simulink model "distributed_UIO_4nodes_switching"  (R2021a)
settings: Solver=VariableStepAuto  StartTime=0.0  StopTime=50  FixedStep=1e-6  RelTol=1e-6
values from neighbouring files (symbols this model uses):
  A = [0,1,0,0,0,0,0,0 ... (first row only)    [UIO_parameters_4nodes_invertedpendulum.m]    (also in UIO_parameters_4nodes_perturbation.m = Xi - diag(sum(Xi,2)); UIO_parameters_4nodes_room_T.m = Xi - diag(sum(Xi,2)); UIO_parameters_4nodes_unknowninputs_directed.m = Xi - diag(sum(Xi,2)); UIO_parameters_4nodes_unknowninputs_switching.m = Xi - diag(sum(Xi,2)))
  B1 = B(:,1)    [UIO_parameters_4nodes_invertedpendulum.m]    (also in UIO_parameters_4nodes_perturbation.m; UIO_parameters_4nodes_room_T.m; UIO_parameters_4nodes_unknowninputs_directed.m; UIO_parameters_4nodes_unknowninputs_switching.m)
  B2 = B(:,2)    [UIO_parameters_4nodes_invertedpendulum.m]    (also in UIO_parameters_4nodes_perturbation.m; UIO_parameters_4nodes_room_T.m; UIO_parameters_4nodes_unknowninputs_directed.m; UIO_parameters_4nodes_unknowninputs_switching.m)
  B3 = B(:,3)    [UIO_parameters_4nodes_invertedpendulum.m]    (also in UIO_parameters_4nodes_perturbation.m; UIO_parameters_4nodes_room_T.m; UIO_parameters_4nodes_unknowninputs_directed.m; UIO_parameters_4nodes_unknowninputs_switching.m)
  C1 = [0,0,0,1,0,0,0,0 ... (first row only)    [UIO_parameters_4nodes_invertedpendulum.m]    (also in UIO_parameters_4nodes_perturbation.m = [0,0,0,0,1,0,0,0,0; UIO_parameters_4nodes_room_T.m = [0,0,0,0,1,0,0,0,0; UIO_parameters_4nodes_unknowninputs_directed.m = [0,0,0,0,1,0,0,0,0; UIO_parameters_4nodes_unknowninputs_switching.m = [0,0,0,0,1,0,0,0,0)
  C2 = [0,1,0,0,0,0,0,0 ... (first row only)    [UIO_parameters_4nodes_invertedpendulum.m]    (also in UIO_parameters_4nodes_perturbation.m = [0,1,0,0,0,0,0,0,0; UIO_parameters_4nodes_room_T.m = [0,1,0,0,0,0,0,0,0; UIO_parameters_4nodes_unknowninputs_directed.m = [0,1,0,0,0,0,0,0,0; UIO_parameters_4nodes_unknowninputs_switching.m = [0,1,0,0,0,0,0,0,0)
  C3 = [0,0,0,1,0,0,0,0 ... (first row only)    [UIO_parameters_4nodes_invertedpendulum.m]    (also in UIO_parameters_4nodes_perturbation.m = [0,1,0,0,0,0,0,0,0; UIO_parameters_4nodes_room_T.m = [0,1,0,0,0,0,0,0,0; UIO_parameters_4nodes_unknowninputs_directed.m = [0,1,0,0,0,0,0,0,0; UIO_parameters_4nodes_unknowninputs_switching.m = [0,1,0,0,0,0,0,0,0)
  C4 = [0,1,0,0,0,0,0,0 ... (first row only)    [UIO_parameters_4nodes_invertedpendulum.m]    (also in UIO_parameters_4nodes_perturbation.m = [0,1,0,0,0,0,0,0,0; UIO_parameters_4nodes_room_T.m = [0,1,0,0,0,0,0,0,0; UIO_parameters_4nodes_unknowninputs_directed.m = [0,1,0,0,0,0,0,0,0; UIO_parameters_4nodes_unknowninputs_switching.m = [0,1,0,0,0,0,0,0,0)
  chi = norm(Lambda + Lambda_P'*(-sum_Lambda)^(-1)*Lambda_P)/(2*lambda_2)+1    [UIO_parameters_4nodes_invertedpendulum.m]    (also in UIO_parameters_4nodes_perturbation.m = norm(Lambda + Lambda_P'*(-sum_Lambda)^(-1)*Lambda_P)/(2*lamb; UIO_parameters_4nodes_room_T.m = norm(Lambda + Lambda_P'*(-sum_Lambda)^(-1)*Lambda_P)/(2*lamb; UIO_parameters_4nodes_unknowninputs_directed.m = norm(Lambda + Lambda_P'*(-sum_Lambda)^(-1)*Lambda_P)/hatLap2; UIO_parameters_4nodes_unknowninputs_switching.m = norm(Lambda + Lambda_P'*(-sum_Lambda)^(-1)*Lambda_P)/(2*CN)+)
  D = B(:,4)    [UIO_parameters_4nodes_invertedpendulum.m]    (also in UIO_parameters_4nodes_perturbation.m; UIO_parameters_4nodes_room_T.m; UIO_parameters_4nodes_unknowninputs_directed.m; UIO_parameters_4nodes_unknowninputs_switching.m)
  F = place(A,[B1,B2,B3],-1*[0.1 0.2 0.3 0.4 0.5 0.6 0.7 0.8])    [UIO_parameters_4nodes_invertedpendulum.m]    (also in UIO_parameters_4nodes_perturbation.m = place(A,[B1,B2,B3],-1*[0.1 0.2 0.3 0.4 0.5 0.6 0.7 0.8 0.9]); UIO_parameters_4nodes_room_T.m = place(A,[B1,B2,B3],-1*[0.1 0.2 0.3 0.4 0.5 0.6 0.7 0.8 0.9]); UIO_parameters_4nodes_unknowninputs_directed.m = place(A,[B1,B2,B3],-1*[0.1 0.2 0.3 0.4 0.5 0.6 0.7 0.8 0.9]); UIO_parameters_4nodes_unknowninputs_switching.m = place(A,[B1,B2,B3],-1*[0.1 0.2 0.3 0.4 0.5 0.6 0.7 0.8 0.9]))
  H1 = U1 + Y1*V1    [UIO_parameters_4nodes_invertedpendulum.m]    (also in UIO_parameters_4nodes_perturbation.m; UIO_parameters_4nodes_room_T.m; UIO_parameters_4nodes_unknowninputs_directed.m; UIO_parameters_4nodes_unknowninputs_switching.m)
  H2 = U2 + Y2*V2    [UIO_parameters_4nodes_invertedpendulum.m]    (also in UIO_parameters_4nodes_perturbation.m; UIO_parameters_4nodes_room_T.m; UIO_parameters_4nodes_unknowninputs_directed.m; UIO_parameters_4nodes_unknowninputs_switching.m)
  H3 = U3 + Y3*V3    [UIO_parameters_4nodes_invertedpendulum.m]    (also in UIO_parameters_4nodes_perturbation.m; UIO_parameters_4nodes_room_T.m; UIO_parameters_4nodes_unknowninputs_directed.m; UIO_parameters_4nodes_unknowninputs_switching.m)
  H4 = U4 + Y4*V4    [UIO_parameters_4nodes_invertedpendulum.m]    (also in UIO_parameters_4nodes_perturbation.m; UIO_parameters_4nodes_room_T.m; UIO_parameters_4nodes_unknowninputs_directed.m; UIO_parameters_4nodes_unknowninputs_switching.m)
  L1 = K1 + N1*H1    [UIO_parameters_4nodes_invertedpendulum.m]    (also in UIO_parameters_4nodes_perturbation.m; UIO_parameters_4nodes_room_T.m; UIO_parameters_4nodes_unknowninputs_directed.m; UIO_parameters_4nodes_unknowninputs_switching.m)
  L2 = K2 + N2*H2    [UIO_parameters_4nodes_invertedpendulum.m]    (also in UIO_parameters_4nodes_perturbation.m; UIO_parameters_4nodes_room_T.m; UIO_parameters_4nodes_unknowninputs_directed.m; UIO_parameters_4nodes_unknowninputs_switching.m)
  L3 = K3 + N3*H3    [UIO_parameters_4nodes_invertedpendulum.m]    (also in UIO_parameters_4nodes_perturbation.m; UIO_parameters_4nodes_room_T.m; UIO_parameters_4nodes_unknowninputs_directed.m; UIO_parameters_4nodes_unknowninputs_switching.m)
  L4 = K4 + N4*H4    [UIO_parameters_4nodes_invertedpendulum.m]    (also in UIO_parameters_4nodes_perturbation.m; UIO_parameters_4nodes_room_T.m; UIO_parameters_4nodes_unknowninputs_directed.m; UIO_parameters_4nodes_unknowninputs_switching.m)
  M1 = eye(n) - H1*C1    [UIO_parameters_4nodes_invertedpendulum.m]    (also in UIO_parameters_4nodes_perturbation.m; UIO_parameters_4nodes_room_T.m; UIO_parameters_4nodes_unknowninputs_directed.m; UIO_parameters_4nodes_unknowninputs_switching.m)
  M2 = eye(n) - H2*C2    [UIO_parameters_4nodes_invertedpendulum.m]    (also in UIO_parameters_4nodes_perturbation.m; UIO_parameters_4nodes_room_T.m; UIO_parameters_4nodes_unknowninputs_directed.m; UIO_parameters_4nodes_unknowninputs_switching.m)
  M3 = eye(n) - H3*C3    [UIO_parameters_4nodes_invertedpendulum.m]    (also in UIO_parameters_4nodes_perturbation.m; UIO_parameters_4nodes_room_T.m; UIO_parameters_4nodes_unknowninputs_directed.m; UIO_parameters_4nodes_unknowninputs_switching.m)
  N1 = M1*A - K1*C1    [UIO_parameters_4nodes_invertedpendulum.m]    (also in UIO_parameters_4nodes_perturbation.m; UIO_parameters_4nodes_room_T.m; UIO_parameters_4nodes_unknowninputs_directed.m; UIO_parameters_4nodes_unknowninputs_switching.m)
  N2 = M2*A - K2*C2    [UIO_parameters_4nodes_invertedpendulum.m]    (also in UIO_parameters_4nodes_perturbation.m; UIO_parameters_4nodes_room_T.m; UIO_parameters_4nodes_unknowninputs_directed.m; UIO_parameters_4nodes_unknowninputs_switching.m)
  N3 = M3*A - K3*C3    [UIO_parameters_4nodes_invertedpendulum.m]    (also in UIO_parameters_4nodes_perturbation.m; UIO_parameters_4nodes_room_T.m; UIO_parameters_4nodes_unknowninputs_directed.m; UIO_parameters_4nodes_unknowninputs_switching.m)
  N4 = M4*A - K4*C4    [UIO_parameters_4nodes_invertedpendulum.m]    (also in UIO_parameters_4nodes_perturbation.m; UIO_parameters_4nodes_room_T.m; UIO_parameters_4nodes_unknowninputs_directed.m; UIO_parameters_4nodes_unknowninputs_switching.m)
  P1 = [0.1 -2.74787163193e-21 -6.58900207734e-22 1.45624208773e-22 2.15066555276e-36 2.0153156439e-36 -1.50571830434e-21 -1.03899300906e-23 2.18840927595e-36 -2.74787163193e-21 0.1 -2.05830389854e-21 ... (81 elements, 9x9)]    [paras_T.mat]
  P2 = [0.1 7.3646299452e-36 -1.12803244841e-21 -8.66266671459e-22 7.23314160582e-22 7.39056861945e-36 -8.2159683555e-21 6.09745804933e-22 7.34683360427e-36 7.3646299452e-36 0.1 1.40040566631e-35 ... (81 elements, 9x9)]    [paras_T.mat]
  P3 = [0.1 -2.18794371664e-37 3.91368207909e-22 3.65670921511e-22 -2.55025634775e-37 -1.42860183838e-23 2.63558676e-21 -2.22685468476e-22 -3.11406679403e-37 -2.18794371664e-37 0.1 -8.43108395867e-38 ... (81 elements, 9x9)]    [paras_T.mat]
  P4 = [0.1 2.36535861574e-35 -1.59743131024e-21 -1.41330471892e-21 2.3619901104e-35 2.36062716781e-35 -1.18359612306e-20 7.3423642543e-22 2.36207112865e-35 2.36535861574e-35 0.1 3.81668075057e-35 ... (81 elements, 9x9)]    [paras_T.mat]
  x0 = -30/180*pi+2*30/180*pi*rand(n,1)    [UIO_parameters_4nodes_invertedpendulum.m]    (also in UIO_parameters_4nodes_perturbation.m = [15.8;27.5;7.4;8.1;11.2;23.2;25.3;23.2;18.3]; UIO_parameters_4nodes_room_T.m = [15.8;27.5;7.4;8.1;11.2;23.2;25.3;23.2;18.3]; UIO_parameters_4nodes_unknowninputs_directed.m = [15.8;27.5;7.4;8.1;11.2;23.2;25.3;23.2;18.3]; UIO_parameters_4nodes_unknowninputs_switching.m = [15.8;27.5;7.4;8.1;11.2;23.2;25.3;23.2;18.3])
  xset = 18*ones(n,1)    [UIO_parameters_4nodes_perturbation.m]    (also in UIO_parameters_4nodes_room_T.m; UIO_parameters_4nodes_unknowninputs_directed.m; UIO_parameters_4nodes_unknowninputs_switching.m; paras_T.mat = [18 18 18 18 18 18 18 18 18])
libraries: simulink x1
settings Model: Creator=gy116  LastModifiedBy=gy116
settings SolverCC: AlgebraicLoopSolver=LineSearch
settings DataIOCC: ReturnWorkspaceOutputs=off
settings DebuggingCC: SFMachineParentedDataDiag=warning  ArithmeticOperatorsInVariantConditions=warning
settings SFSimCC: SimUseLocalCustomCode=off  CustomCodeUndefinedFunction=UseInterfaceOnly
settings RTWCC: RTWUseLocalCustomCode=off
settings CodeAppCC: StateflowObjectComments=on

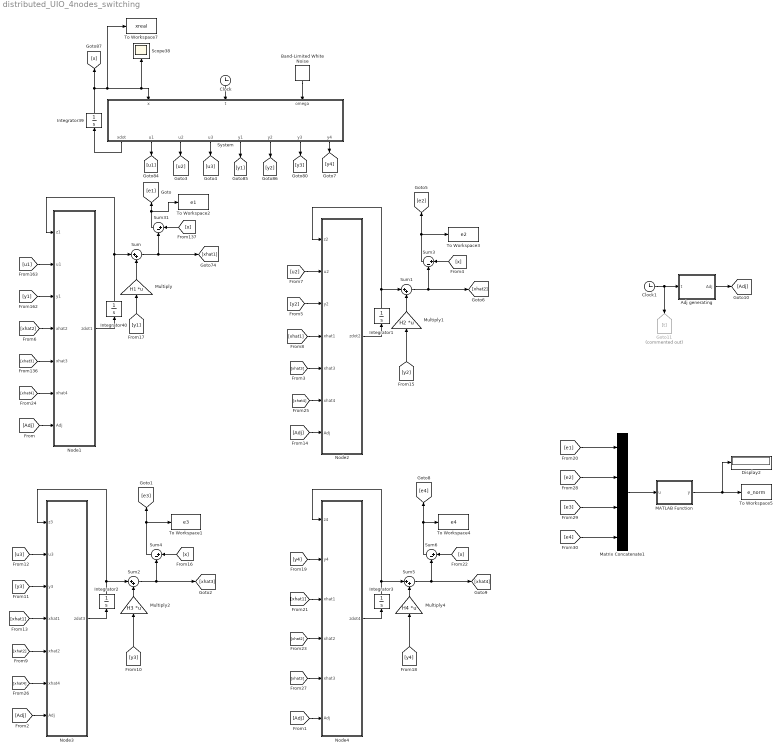
== system distributed_UIO_4nodes_switching ==
  Adj generating : MATLAB Function  TreatAsAtomicUnit=on
  Band-Limited White Noise : simulink/Sources/Band-Limited White Noise  Cov=[1]  Ts=0.1  seed=[23341]
  Clock : Clock
  Clock1 : Clock
  Display2 : Display
  Goto11 : Goto  Commented=on  GotoTag=t
  Integrator{1..3,40} (4 alike) : Integrator  InitialCondition=0*x0
  Integrator39 : Integrator  InitialCondition=x0
  MATLAB Function : MATLAB Function  TreatAsAtomicUnit=on
  Matrix Concatenate1 : Concatenate  NumInputs=4  ConcatenateDimension=2
  Multiply : Gain  Gain=H1  Multiplication=Matrix(K*u) (u vector)
  Multiply1 : Gain  Gain=H2  Multiplication=Matrix(K*u) (u vector)
  Multiply2 : Gain  Gain=H3  Multiplication=Matrix(K*u) (u vector)
  Multiply4 : Gain  Gain=H4  Multiplication=Matrix(K*u) (u vector)
  Node1 : MATLAB Function  TreatAsAtomicUnit=on
  Node2 : MATLAB Function  TreatAsAtomicUnit=on
  Node3 : MATLAB Function  TreatAsAtomicUnit=on
  Node4 : MATLAB Function  TreatAsAtomicUnit=on
  Scope38 : Scope
  Sum{,1..2,5} (4 alike) : Sum  Inputs=|++
  Sum{3..4,6,31} (4 alike) : Sum  Inputs=|+-
  System : MATLAB Function  TreatAsAtomicUnit=on
  To Workspace1 : ToWorkspace  VariableName=e3  SaveFormat=Structure With Time  SampleTime=-1
  To Workspace2 : ToWorkspace  VariableName=e1  SaveFormat=Structure With Time  SampleTime=-1
  To Workspace3 : ToWorkspace  VariableName=e2  SaveFormat=Structure With Time  SampleTime=-1
  To Workspace4 : ToWorkspace  VariableName=e4  SaveFormat=Structure With Time  SampleTime=-1
  To Workspace5 : ToWorkspace  VariableName=e_norm  SaveFormat=Structure With Time  SampleTime=-1
  To Workspace7 : ToWorkspace  VariableName=xreal  SaveFormat=Structure With Time  SampleTime=-1
  wires:
  Clock1/1 -> Adj generating/1(t), Goto11/1
  Adj generating/1(Adj) -> [Adj]
  [x] -> Sum6/1
  Integrator40/1 -> Sum/1, Node1/1(z1)
  [xhat1] -> Node3/4(xhat1)
  Sum6/1 -> To Workspace4/1, [e4]
  Multiply4/1 -> Sum5/2
  Integrator3/1 -> Sum5/1, Node4/1(z4)
  Node1/1(zdot1) -> Integrator40/1
  [y1] -> Node1/3(y1)
  Sum2/1 -> Sum4/2, [xhat3]
  [y1] -> Multiply/1
  [y3] -> Multiply2/1
  [y2] -> Multiply1/1
  Sum/1 -> Sum31/2, [xhat1]
  Node4/1(zdot4) -> Integrator3/1
  Integrator39/1 -> To Workspace7/1, System/1(x), Scope38/1, [x]
  Band-Limited White Noise/1 -> System/3(omega)
  [u3] -> Node3/2(u3)
  [y4] -> Multiply4/1
  Sum1/1 -> Sum3/2, [xhat2]
  [xhat4] -> Node2/6(xhat4)
  System/8(y4) -> [y4]
  System/5(y1) -> [y1]
  [y4] -> Node4/2(y4)
  [xhat2] -> Node4/4(xhat2)
  [xhat3] -> Node4/5(xhat3)
  Multiply1/1 -> Sum1/2
  Sum3/1 -> To Workspace3/1, [e2]
  System/1(xdot) -> Integrator39/1
  System/3(u2) -> [u2]
  Clock/1 -> System/2(t)
  [xhat2] -> Node1/4(xhat2)
  System/7(y3) -> [y3]
  [x] -> Sum31/1
  System/2(u1) -> [u1]
  Integrator1/1 -> Sum1/1, Node2/1(z2)
  [xhat4] -> Node3/6(xhat4)
  [y2] -> Node2/3(y2)
  [y3] -> Node3/3(y3)
  Integrator2/1 -> Sum2/1, Node3/1(z3)
  Sum31/1 -> To Workspace2/1, [e1]
  [xhat3] -> Node2/5(xhat3)
  [u2] -> Node2/2(u2)
  [xhat2] -> Node3/5(xhat2)
  Multiply/1 -> Sum/2
  System/6(y2) -> [y2]
  [xhat3] -> Node1/5(xhat3)
  [x] -> Sum3/1
  Node2/1(zdot2) -> Integrator1/1
  Node3/1(zdot3) -> Integrator2/1
  [x] -> Sum4/1
  [u1] -> Node1/2(u1)
  [xhat1] -> Node2/4(xhat1)
  Sum4/1 -> To Workspace1/1, [e3]
  System/4(u3) -> [u3]
  Sum5/1 -> Sum6/2, [xhat4]
  [xhat1] -> Node4/3(xhat1)
  Multiply2/1 -> Sum2/2
  [xhat4] -> Node1/6(xhat4)
  [Adj] -> Node1/7(Adj)
  [Adj] -> Node2/7(Adj)
  [Adj] -> Node3/7(Adj)
  [Adj] -> Node4/6(Adj)
  [e4] -> Matrix Concatenate1/4
  Matrix Concatenate1/1 -> MATLAB Function/1(u)
  [e1] -> Matrix Concatenate1/1
  [e3] -> Matrix Concatenate1/3
  MATLAB Function/1(y) -> Display2/1, To Workspace5/1
  [e2] -> Matrix Concatenate1/2

== matlab function distributed_UIO_4nodes_switching/MATLAB Function ==
  data: u input; y output
function y = fcn(u)

y = norm(u);

== matlab function distributed_UIO_4nodes_switching/Node1 ==
  data: z1 input; u1 input; y1 input; xhat2 input; xhat3 input; xhat4 input; zdot1 output; N1 parameter; M1 parameter; L1 parameter; P1 parameter; B1 parameter; H1 parameter; chi parameter; Adj input
function zdot1  = fcn(z1,u1,y1,xhat2,xhat3,xhat4,N1, M1, L1, P1,B1, H1, chi, Adj)

commu1 =  Adj(1,2)*(xhat2-z1-H1*y1) + Adj(1,3)*(xhat3-z1-H1*y1) + Adj(1,4)*(xhat4-z1-H1*y1);

zdot1 = N1*z1 + M1*B1*u1 + L1*y1 + chi*P1^(-1)*commu1;

== matlab function distributed_UIO_4nodes_switching/System ==
  data: x input; t input; A parameter; xdot output; u1 output; u2 output; u3 output; y1 output; y2 output; y3 output; B1 parameter; B2 parameter; B3 parameter; C2 parameter; C3 parameter; C1 parameter; F parameter; omega input; y4 output; D parameter; C4 parameter; xset parameter
function [xdot,u1,u2,u3,y1,y2,y3,y4] = fcn(x,t,A,B1,B2,B3,C2, C3, C1,F,omega, D, C4,xset)
u = [-F*(x-xset);omega];
xdot = A*x + [B1,B2,B3,D]*u;

u1 = u(1);
u2 = u(2);
u3 = u(3);
% u4 = [u1;u2;u3];

y1 = C1*x;
y2 = C2*x;
y3 = C3*x;
y4 = C4*x;

== matlab function distributed_UIO_4nodes_switching/Node2 ==
  data: z2 input; u2 input; y2 input; xhat1 input; xhat3 input; xhat4 input; zdot2 output; N2 parameter; M2 parameter; L2 parameter; P2 parameter; chi parameter; B2 parameter; H2 parameter; Adj input
function zdot2   = fcn(z2,u2,y2,xhat1,xhat3,xhat4,N2, M2, L2, P2,chi, B2, H2, Adj)

commu2 =  Adj(2,1)*(xhat1-z2-H2*y2) + Adj(2,3)*(xhat3-z2-H2*y2) + Adj(2,4)*(xhat4-z2-H2*y2);

zdot2 = N2*z2 + M2*B2*u2 + L2*y2 + chi*P2^(-1)*commu2;
% xhat2 = z2 - E2*y2;

== matlab function distributed_UIO_4nodes_switching/Node3 ==
  data: z3 input; u3 input; y3 input; xhat1 input; xhat2 input; xhat4 input; zdot3 output; N3 parameter; M3 parameter; L3 parameter; P3 parameter; chi parameter; H3 parameter; B3 parameter; Adj input
function zdot3   = fcn(z3,u3,y3,xhat1,xhat2,xhat4,N3, M3, L3, P3,chi, H3, B3, Adj)

commu3 =  Adj(3,1)*(xhat1-z3-H3*y3) + Adj(3,2)*(xhat2-z3-H3*y3) + + Adj(3,4)*(xhat4-z3-H3*y3);

zdot3 = N3*z3 + M3*B3*u3 + L3*y3 + chi*P3^(-1)*commu3;
% xhat3 = z3 - E3*y3;

== matlab function distributed_UIO_4nodes_switching/Node4 ==
  data: z4 input; y4 input; xhat1 input; xhat2 input; xhat3 input; zdot4 output; N4 parameter; L4 parameter; P4 parameter; chi parameter; H4 parameter; Adj input
function zdot4   = fcn(z4,y4,xhat1,xhat2,xhat3,N4,L4, P4,chi, H4, Adj)

commu4 =  Adj(4,1)*(xhat1-z4-H4*y4) + Adj(4,2)*(xhat2-z4-H4*y4) + Adj(4,3)*(xhat3-z4-H4*y4);

% zdot4 = N4*z4 + G4*u4+ L4*y4 + chi*P4^(-1)*commu4;
zdot4 = N4*z4 + L4*y4 + chi*P4^(-1)*commu4;
% xhat4 = z4 - E4*y4;

== matlab function distributed_UIO_4nodes_switching/Adj generating ==
  data: t input; Adj output
function Adj = fcn(t)
t = t/0.1;
tik = mod(t,4);
if (tik>=0) && (tik<1)
    Adj = [0,1,1,1;
           1,0,0,1;
           1,0,0,1;
           1,1,1,0];
elseif (tik>=1) && (tik<2)
    Adj = [0,1,0,0;
           1,0,0,1;
           0,0,0,1;
           0,1,1,0];
elseif (tik>=2) && (tik<3)
    Adj = [0,1,0,0;
           1,0,1,1;
           0,1,0,0;
           0,1,0,0];
elseif (tik>=3) && (tik<4)
    Adj = [0,1,1,0;
           1,0,0,0;
           1,0,0,1;
           0,0,1,0];
else
    Adj = zeros(4,4);
end
end
